simulink model "MDCC"  (R2021b)
settings: Solver=FixedStepDiscrete  StartTime=0.0  StopTime=10.0  FixedStep=0.0001  RelTol=1e-3
model workspace (MATLAB code in the model file):
  | cmdLim = Simulink.Parameter;
  | cmdLim.Value = 15;
  | cmdLim.Description = 'Limit for controlling the maximum surface command angle.';
  | cmdLim.Min = 0;
  | cmdLim.Max = 90;
  | cmdLim.DocUnits = 'deg';
  | 
  | dispGain = Simulink.Parameter;
  | dispGain.Value = 0.75;
  | dispGain.Description = 'Gain applied to the displacement error.';
  | dispGain.Min = 0;
  | dispGain.Max = [];
  | dispGain.DocUnits = 'deg/sec/deg';
  | 
  | dispLim = Simulink.Parameter;
  | dispLim.Value = 30;
  | dispLim.Description = 'Limit for controlling the maximum commanded angle.';
  | dispLim.Min = 0;
  | dispLim.Max = 180;
  | dispLim.DocUnits = 'deg';
  | 
  | intGain = Simulink.Parameter;
  | intGain.Value = 0.5;
  | intGain.Description = 'Gain applied to the integral error.';
  | intGain.Min = 0;
  | intGain.Max = [];
  | intGain.DocUnits = 'deg/sec/deg/sec';
  | 
  | intLim = Simulink.Parameter;
  | intLim.Value = 5;
  | intLim.Description = 'Limit for controlling the maximum commanded angle.';
  | intLim.Min = 0;
  | intLim.Max = 90;
  | intLim.DocUnits = 'deg';
  | 
  | rateGain = Simulink.Parameter;
  | rateGain.Value = 2;
  | rateGain.Description = 'Gain applied to the rate error.';
  | rateGain.Min = 0;
  | rateGain.Max = [];
  | rateGain.DocUnits = 'deg/deg/sec';
  | 
  | rateLim = Simulink.Parameter;
  | rateLim.Value = 6;
  | rateLim.Description = 'Limit for controlling the maximum commanded angle.';
  | rateLim.Min = 0;
  | rateLim.Max = 180;
  | rateLim.DocUnits = 'deg/sec';
  | 
  | hdgGain = Simulink.Parameter;
  | hdgGain.Value = 0.015;
values from neighbouring files (symbols this model uses):
  KfDeadCompen_SetDeltaTime_us = myPackage.Parameter    [DeadCompen.m]
  Ts = 5E-6    (= 5e-06)    [iPMSM_data.m]
  VbDeadComp_SwtUseIsttrDes_flg = myPackage.Parameter    [DeadCompen.m]
  VfDeadCompen_ISttrDdeThdSwt_A = myPackage.Parameter    [DeadCompen.m]
  VfDeadCompen_ISttrIgbtThdSwt_A = myPackage.Parameter    [DeadCompen.m]
  VfDeadCompen_rDdeISttrHi_R = myPackage.Parameter    [DeadCompen.m]
  VfDeadCompen_rDdeISttrLo_R = myPackage.Parameter    [DeadCompen.m]
  VfDeadCompen_rIgbtISttrHi_R = myPackage.Parameter    [DeadCompen.m]
  VfDeadCompen_rIgbtISttrLo_R = myPackage.Parameter    [DeadCompen.m]
  VfDeadCompen_uDdeISttrHi_V = myPackage.Parameter    [DeadCompen.m]
  VfDeadCompen_uDdeISttrLo_V = myPackage.Parameter    [DeadCompen.m]
  VfDeadCompen_uIgbtISttrHi_V = myPackage.Parameter    [DeadCompen.m]
  VfDeadCompen_uIgbtISttrLo_V = myPackage.Parameter    [DeadCompen.m]
undefined symbols (not defined in the file or in its folder): CosTable12bit_Y, GLBCal_GLBCal_Kf_DCLinkOverVolErrThd_V, GLBCal_GLBCal_Kf_DCLinkUnderVolErrThd_V, GLBCal_GLBCal_Kf_EquiLd_NULL, GLBCal_GLBCal_Kf_EquiLq_NULL, GLBCal_GLBCal_Kf_MotorRatedSpeed_rpm, GLBCal_GLBCal_Kf_MotorSpeedHysteresis_Coef, GLBCal_Ke_MotorPolePairsNum_NULL, IoHwAbOpArg_PwmDutyCyclePhU_NULL, IoHwAbOpArg_PwmDutyCyclePhV_NULL, IoHwAbOpArg_PwmDutyCyclePhW_NULL, IoHwAbOpArg_PwmOutputEn, KbMDCC_DeadTimeCompEn_flg, KbMDCC_MCF_flgHarmInIsdqTab11ZR_flg, KbMDCC_MCF_flgHarmInIsdqTab13ZR_flg, KbMDCC_MCF_flgHarmInIsdqTab5ZR_flg, KbMDCC_MCF_flgHarmInIsdqTab7ZR_flg, KbMDCC_MCF_flgHarmInject_flg, KbMDCC_SetEAngleEn_flg, KbMDCC_UdUqFwOmit_flg, KfDeadCompen_CpPeriodTimesT_NULL, KfMDCC_ActiveDischargeIdCurVal_A, KfMDCC_ActiveDischargeIqCurVal_A, KfMDCC_DCLinkVolRate_coef, KfMDCC_DebugEAngleInit_rad, KfMDCC_DebugUalphaVolCmd_V, KfMDCC_DebugUbetaVolCmd_V, KfMDCC_DebugUdCmd_V, KfMDCC_DebugUqCmd_V, KfMDCC_DebugUsCmd_V, KfMDCC_DebugUsRate_V, KfMDCC_IMCResp_NULL, KfMDCC_IMCStab_NULL, KfMDCC_InvParkCpPeriodTimesT_NULL, KfMDCC_MCF_CircAge_NULL, KfMDCC_MCF_flgUse11Harm_flg, KfMDCC_MCF_flgUse13Harm_flg, KfMDCC_MCF_flgUse5Harm_flg, KfMDCC_MCF_flgUse7Harm_flg, KfMDCC_MCF_Harm1113FLParamSpeedThrd_rads, KfMDCC_MCF_Harm57FLParamSpeedThrd_rads, KfMDCC_MCF_HarmcofFltN_NULL, KfMDCC_MCF_HarmCpnAg_NULL, KfMDCC_MCF_HarmfLParaHigh_coef, KfMDCC_MCF_HarmfLParaLow_coef, KfMDCC_MCF_HarmIn1113ZRY_Trq_Nm, KfMDCC_MCF_HarmIn11_SpdLimHigh_rads, KfMDCC_MCF_HarmIn11_SpdLimLow_rads, KfMDCC_MCF_HarmIn11ZRY_Isd_A, KfMDCC_MCF_HarmIn11ZRY_Isq_A, KfMDCC_MCF_HarmIn13_SpdLimHigh_rads, KfMDCC_MCF_HarmIn13_SpdLimLow_rads, KfMDCC_MCF_HarmIn13ZRY_Isd_A, KfMDCC_MCF_HarmIn13ZRY_Isq_A, KfMDCC_MCF_HarmIn57ZRY_Trq_Nm, KfMDCC_MCF_HarmIn5_SpdLimHigh_rads, KfMDCC_MCF_HarmIn5_SpdLimLow_rads, KfMDCC_MCF_HarmIn5ZRY_Isd_A, KfMDCC_MCF_HarmIn5ZRY_Isq_A, KfMDCC_MCF_HarmIn7_SpdLimHigh_rads ... (+47)
libraries: simulink x40, PMSM_Library x3, mcbcontrolslib x1
(part 4 of 8)

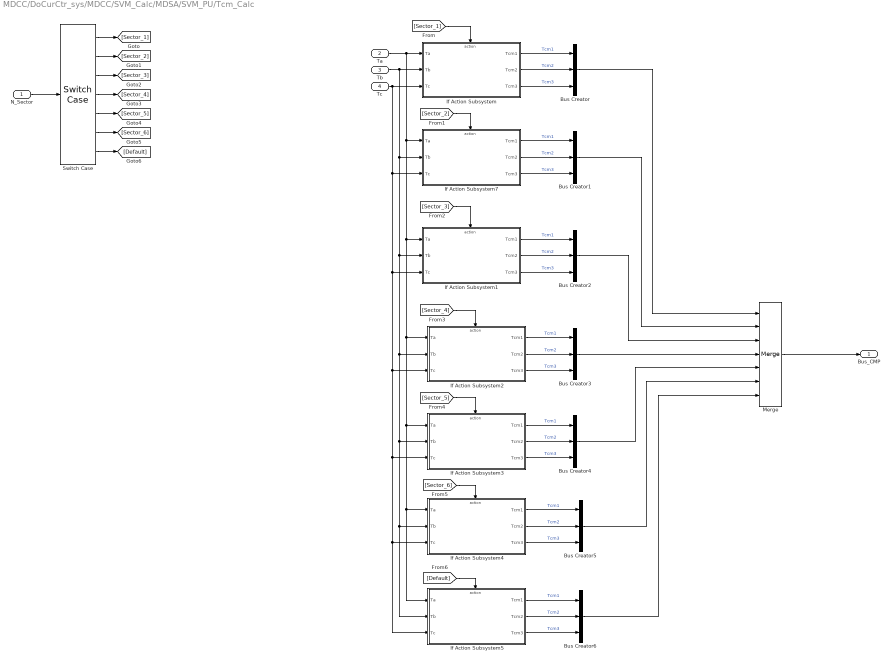
== system MDCC/DoCurCtr_sys/MDCC/SVM_Calc/MDSA/SVM_PU/Tcm_Calc ==
  N_Sector : Inport
  Ta : Inport  Port=2
  Tb : Inport  Port=3
  Tc : Inport  Port=4
  Bus Creator{,1..6} (7 alike) : BusCreator  Inputs=3
  If Action Subsystem : Subsystem  TreatAsAtomicUnit=on
  If Action Subsystem1 : Subsystem  TreatAsAtomicUnit=on
  If Action Subsystem2 : Subsystem  TreatAsAtomicUnit=on
  If Action Subsystem3 : Subsystem  TreatAsAtomicUnit=on
  If Action Subsystem4 : Subsystem  TreatAsAtomicUnit=on
  If Action Subsystem5 : Subsystem  TreatAsAtomicUnit=on
  If Action Subsystem7 : Subsystem  TreatAsAtomicUnit=on
  Merge : Merge  Inputs=7
  Switch Case : SwitchCase  CaseConditions={1,2,3,4,5,6}
  Bus_CMP : Outport
  wires:
  Switch Case/1 -> [Sector_1]
  Switch Case/2 -> [Sector_2]
  Switch Case/4 -> [Sector_4]
  Switch Case/6 -> [Sector_6]
  Switch Case/3 -> [Sector_3]
  N_Sector/1 -> Switch Case/1
  Switch Case/7 -> [Default]
  Switch Case/5 -> [Sector_5]
  [Sector_1] -> If Action Subsystem/Action
  [Sector_2] -> If Action Subsystem7/Action
  [Sector_4] -> If Action Subsystem2/Action
  [Sector_3] -> If Action Subsystem1/Action
  [Sector_6] -> If Action Subsystem4/Action
  [Sector_5] -> If Action Subsystem3/Action
  [Default] -> If Action Subsystem5/Action
  Tb/1 -> If Action Subsystem5/2(Tb), If Action Subsystem4/2(Tb), If Action Subsystem3/2(Tb), If Action Subsystem2/2(Tb), If Action Subsystem1/2(Tb), If Action Subsystem7/2(Tb), If Action Subsystem/2(Tb)
  Tc/1 -> If Action Subsystem/3(Tc), If Action Subsystem5/3(Tc), If Action Subsystem4/3(Tc), If Action Subsystem3/3(Tc), If Action Subsystem2/3(Tc), If Action Subsystem1/3(Tc), If Action Subsystem7/3(Tc)
  Ta/1 -> If Action Subsystem5/1(Ta), If Action Subsystem4/1(Ta), If Action Subsystem3/1(Ta), If Action Subsystem2/1(Ta), If Action Subsystem1/1(Ta), If Action Subsystem7/1(Ta), If Action Subsystem/1(Ta)
  Merge/1 -> Bus_CMP/1
  If Action Subsystem/1(Tcm1) -> Bus Creator/1  "Tcm1"
  If Action Subsystem/2(Tcm2) -> Bus Creator/2  "Tcm2"
  If Action Subsystem/3(Tcm3) -> Bus Creator/3  "Tcm3"
  If Action Subsystem7/1(Tcm1) -> Bus Creator1/1  "Tcm1"
  If Action Subsystem7/3(Tcm3) -> Bus Creator1/3  "Tcm3"
  If Action Subsystem7/2(Tcm2) -> Bus Creator1/2  "Tcm2"
  If Action Subsystem1/1(Tcm1) -> Bus Creator2/1  "Tcm1"
  If Action Subsystem1/3(Tcm3) -> Bus Creator2/3  "Tcm3"
  If Action Subsystem1/2(Tcm2) -> Bus Creator2/2  "Tcm2"
  If Action Subsystem2/1(Tcm1) -> Bus Creator3/1  "Tcm1"
  If Action Subsystem2/3(Tcm3) -> Bus Creator3/3  "Tcm3"
  If Action Subsystem2/2(Tcm2) -> Bus Creator3/2  "Tcm2"
  If Action Subsystem3/1(Tcm1) -> Bus Creator4/1  "Tcm1"
  If Action Subsystem3/3(Tcm3) -> Bus Creator4/3  "Tcm3"
  If Action Subsystem3/2(Tcm2) -> Bus Creator4/2  "Tcm2"
  If Action Subsystem4/1(Tcm1) -> Bus Creator5/1  "Tcm1"
  If Action Subsystem4/3(Tcm3) -> Bus Creator5/3  "Tcm3"
  If Action Subsystem4/2(Tcm2) -> Bus Creator5/2  "Tcm2"
  If Action Subsystem5/1(Tcm1) -> Bus Creator6/1  "Tcm1"
  If Action Subsystem5/3(Tcm3) -> Bus Creator6/3  "Tcm3"
  If Action Subsystem5/2(Tcm2) -> Bus Creator6/2  "Tcm2"
  Bus Creator/1 -> Merge/1
  Bus Creator1/1 -> Merge/2
  Bus Creator2/1 -> Merge/3
  Bus Creator3/1 -> Merge/4
  Bus Creator4/1 -> Merge/5
  Bus Creator5/1 -> Merge/6
  Bus Creator6/1 -> Merge/7

== system MDCC/DoCurCtr_sys/MDCC/SVM_Calc/MDSA/SVPWM/vIntp_PWMFOC_CalSec ==
  Bus_UalphaUbeta : Inport
  CalABC : Subsystem
  CalSecValue : Subsystem
  CalVaVbVc : Subsystem  TreatAsAtomicUnit=on
  SecValue : Outport
  N_VALUE : Outport  Port=2
  wires:
  CalSecValue/2(N_VALUE) -> N_VALUE/1
  Bus_UalphaUbeta/1 -> CalVaVbVc/1(Bus_UalphaUbeta)
  CalSecValue/1(SecValue) -> SecValue/1
  CalABC/1(Bus_ABC) -> CalSecValue/1(Bus_ABC_IN)
  CalVaVbVc/1(Bus_Vabc) -> CalABC/1(Bus_Vabc_IN)

== system MDCC/DoCurCtr_sys/MDCC/SVM_Calc/MDSA/SVPWM/vIntp_PWMFOC_CalTriCompValue ==
  note: // 需要确定PWM的passive level
  N_VALUE_IN : Inport
  Bus_UalphaUbeta : Inport  Port=2
  Bus_Ts_Vdc : Inport  Port=3
  CalCMPValue : Subsystem
  CalTabc : Subsystem
  CalXYZ : Subsystem
  Bus_CMP : Outport
  wires:
  Bus_Ts_Vdc/1 -> CalXYZ/2(Bus_Ts_Vdc), CalTabc/2(Bus_Ts_Vdc)
  CalCMPValue/1(Bus_CMP) -> Bus_CMP/1
  CalTabc/1(Bus_Tabc) -> CalCMPValue/1(Bus_Tabc_IN)
  CalXYZ/1(BUS_XYZ) -> CalTabc/1(Bus_XYZ_IN)
  Bus_UalphaUbeta/1 -> CalXYZ/1(Bus_UalphaUbeta)
  N_VALUE_IN/1 -> CalCMPValue/2(N_VALUE_IN), CalTabc/3(N_VALUE_IN)

== system MDCC/DoCurCtr_sys/MDCC/UdUqCalc_Sys/MDCC_MCF_Sys/Enabled Subsystem/Harmonic_Injection_11 ==
  note: 扭矩滞环
  TDC_TrqDes : Inport
  MCF_Harm_isdAct11 : Inport  Port=2
  MCF_Harm_isqAct11 : Inport  Port=3
  MCF_Sin11Ag : Inport  Port=4
  MCF_Cos11Ag : Inport  Port=5
  Rdc_absnWoFlt_rads : Inport  Port=6
  MCF_uDcLnk : Inport  Port=7
  Bus Creator : BusCreator  Inputs=2
  Bus Creator1 : BusCreator  Inputs=2
  Bus Selector : BusSelector  OutputSignals=MCF_uAlpha_Harm11,MCF_uBeta_Harm11
  Set_11_steps_current_isdqdes : Subsystem
  Signal Copy : SignalConversion  OverrideOpt=off
  Signal Copy1 : SignalConversion  OverrideOpt=off
  Subsystem : Subsystem
  Subsystem1 : Subsystem
  Subsystem2 : Subsystem
  Switch2 : Switch  Criteria=u2 ~= 0
  Unit Delay : UnitDelay  SampleTime=-1  HasFrameUpgradeWarning=on
  Zero : Constant  Value=0  OutDataTypeStr=single
  Zero1 : Constant  Value=0  OutDataTypeStr=single
  MCF_uAlpha_Harm11 : Outport
  MCF_uBeta_Harm11 : Outport  Port=2
  wires:
  Bus Selector/2 -> Signal Copy1/1  "<MCF_uBeta_Harm11>"
  Subsystem/1(MCF_uAlpha_Harm11) -> Bus Creator/1  "MCF_uAlpha_Harm11"
  Zero1/1 -> Bus Creator1/2  "MCF_uBeta_Harm11"
  Switch2/1 -> Bus Selector/1
  Bus Creator/1 -> Switch2/1
  Bus Creator1/1 -> Switch2/3
  Zero/1 -> Bus Creator1/1  "MCF_uAlpha_Harm11"
  Subsystem/2(MCF_uBeta_Harm11) -> Bus Creator/2  "MCF_uBeta_Harm11"
  Bus Selector/1 -> Signal Copy/1  "<MCF_uAlpha_Harm11>"
  Subsystem1/1(Out2) -> Subsystem/Enable, Switch2/2, [flgHarmUse], Unit Delay/1
  Signal Copy/1 -> MCF_uAlpha_Harm11/1  "VAR_MCF_uAlpha_Harm11_f32"
  Signal Copy1/1 -> MCF_uBeta_Harm11/1  "VAR_MCF_uBeta_Harm11_f32"
  MCF_Harm_isdAct11/1 -> Subsystem/3(MCF_Harm_isdAct11)
  MCF_Harm_isqAct11/1 -> Subsystem/4(MCF_Harm_isqAct11)
  Unit Delay/1 -> Subsystem/8(MCF_flgHarm11PIRest)
  MCF_Sin11Ag/1 -> Subsystem/5(MCF_Sin11Ag)
  MCF_Cos11Ag/1 -> Subsystem/6(MCF_Cos11Ag)
  Rdc_absnWoFlt_rads/1 -> Subsystem1/1(Rdc_absnWoFlt_rads), Subsystem/7(Rdc_absnWoFlt_rads)
  Set_11_steps_current_isdqdes/1(VfMDCC_MCF_IsdDes11Harm_A) -> Subsystem/1(MCF_Harm_isdDes11)
  Set_11_steps_current_isdqdes/2(VfMDCC_MCF_IsqDes11Harm_A) -> Subsystem/2(MCF_Harm_isqDes11)
  TDC_TrqDes/1 -> Subsystem2/1(TDC_TrqDes)
  Subsystem2/1(TDC_TrqDesFlt) -> Set_11_steps_current_isdqdes/1(TDC_TrqDesFlt)
  [flgHarmUse] -> Subsystem2/2(flgHarmUse)
  MCF_uDcLnk/1 -> Subsystem1/2(MCF_uDcLnk)

== system MDCC/DoCurCtr_sys/MDCC/UdUqCalc_Sys/MDCC_MCF_Sys/Enabled Subsystem/Harmonic_Injection_13 ==
  note: 扭矩滞环
  TDC_TrqDes : Inport
  MCF_Harm_isdAct13 : Inport  Port=2
  MCF_Harm_isqAct13 : Inport  Port=3
  MCF_Sin13Ag : Inport  Port=4
  MCF_Cos13Ag : Inport  Port=5
  Rdc_absnWoFlt_rads : Inport  Port=6
  MCF_uDcLnk : Inport  Port=7
  Bus Creator : BusCreator  Inputs=2
  Bus Creator1 : BusCreator  Inputs=2
  Bus Selector : BusSelector  OutputSignals=MCF_uAlpha_Harm13,MCF_uBeta_Harm13
  Set_13_steps_current_isdqdes : Subsystem
  Signal Copy : SignalConversion  OverrideOpt=off
  Signal Copy1 : SignalConversion  OverrideOpt=off
  Subsystem : Subsystem
  Subsystem1 : Subsystem
  Subsystem2 : Subsystem
  Switch2 : Switch  Criteria=u2 ~= 0
  Unit Delay : UnitDelay  SampleTime=-1  HasFrameUpgradeWarning=on
  Zero : Constant  Value=0  OutDataTypeStr=single
  Zero1 : Constant  Value=0  OutDataTypeStr=single
  MCF_uAlpha_Harm13 : Outport
  MCF_uBeta_Harm13 : Outport  Port=2
  wires:
  Bus Selector/2 -> Signal Copy1/1  "<MCF_uBeta_Harm13>"
  Subsystem/1(MCF_uAlpha_Harm13) -> Bus Creator/1  "MCF_uAlpha_Harm13"
  Zero1/1 -> Bus Creator1/2  "MCF_uBeta_Harm13"
  Switch2/1 -> Bus Selector/1
  Bus Creator/1 -> Switch2/1
  Bus Creator1/1 -> Switch2/3
  Zero/1 -> Bus Creator1/1  "MCF_uAlpha_Harm13"
  Subsystem/2(MCF_uBeta_Harm13) -> Bus Creator/2  "MCF_uBeta_Harm13"
  Bus Selector/1 -> Signal Copy/1  "<MCF_uAlpha_Harm13>"
  Subsystem1/1(Out2) -> Subsystem/Enable, Switch2/2, [flgHarmUse], Unit Delay/1
  Signal Copy/1 -> MCF_uAlpha_Harm13/1  "VAR_MCF_uAlpha_Harm13_f32"
  Signal Copy1/1 -> MCF_uBeta_Harm13/1  "VAR_MCF_uBeta_Harm13_f32"
  MCF_Harm_isdAct13/1 -> Subsystem/3(MCF_Harm_isdAct13)
  MCF_Harm_isqAct13/1 -> Subsystem/4(MCF_Harm_isqAct13)
  Unit Delay/1 -> Subsystem/8(MCF_flgHarm13PIRest)
  MCF_Sin13Ag/1 -> Subsystem/5(MCF_Sin13Ag)
  MCF_Cos13Ag/1 -> Subsystem/6(MCF_Cos13Ag)
  Rdc_absnWoFlt_rads/1 -> Subsystem1/1(Rdc_absnWoFlt_rads), Subsystem/7(Rdc_absnWoFlt_rads)
  Set_13_steps_current_isdqdes/1(VfMDCC_MCF_IsdDes13Harm_A) -> Subsystem/1(MCF_Harm_isdDes13)
  Set_13_steps_current_isdqdes/2(VfMDCC_MCF_IsqDes13Harm_A) -> Subsystem/2(MCF_Harm_isqDes13)
  TDC_TrqDes/1 -> Subsystem2/1(TDC_TrqDes)
  Subsystem2/1(TDC_TrqDesFlt) -> Set_13_steps_current_isdqdes/1(TDC_TrqDesFlt)
  [flgHarmUse] -> Subsystem2/2(flgHarmUse)
  MCF_uDcLnk/1 -> Subsystem1/2(MCF_uDcLnk)

== system MDCC/DoCurCtr_sys/MDCC/UdUqCalc_Sys/MDCC_MCF_Sys/Enabled Subsystem/Harmonic_Injection_5 ==
  note: 扭矩滞环
  TDC_TrqDes : Inport
  MCF_Harm_isdAct5 : Inport  Port=2
  MCF_Harm_isqAct5 : Inport  Port=3
  MCF_Sin5Ag : Inport  Port=4
  MCF_Cos5Ag : Inport  Port=5
  Rdc_absnWoFlt_rads : Inport  Port=6
  MCF_uDcLnk : Inport  Port=7
  Bus Creator : BusCreator  Inputs=2
  Bus Creator1 : BusCreator  Inputs=2
  Bus Selector : BusSelector  OutputSignals=MCF_uAlpha_Harm5,MCF_uBeta_Harm5
  Set_5_steps_current_isdqdes : Subsystem
  Signal Copy : SignalConversion  OverrideOpt=off
  Signal Copy1 : SignalConversion  OverrideOpt=off
  Subsystem : Subsystem
  Subsystem1 : Subsystem
  Subsystem2 : Subsystem
  Switch2 : Switch  Criteria=u2 ~= 0
  Unit Delay : UnitDelay  SampleTime=-1  HasFrameUpgradeWarning=on
  Zero : Constant  Value=0  OutDataTypeStr=single
  Zero1 : Constant  Value=0  OutDataTypeStr=single
  MCF_uAlpha_Harm5 : Outport
  MCF_uBeta_Harm5 : Outport  Port=2
  wires:
  Bus Selector/2 -> Signal Copy1/1  "<MCF_uBeta_Harm5>"
  Subsystem/1(MCF_uAlpha_Harm5) -> Bus Creator/1  "MCF_uAlpha_Harm5"
  Zero1/1 -> Bus Creator1/2  "MCF_uBeta_Harm5"
  Switch2/1 -> Bus Selector/1
  Bus Creator/1 -> Switch2/1
  Bus Creator1/1 -> Switch2/3
  Zero/1 -> Bus Creator1/1  "MCF_uAlpha_Harm5"
  Subsystem/2(MCF_uBeta_Harm5) -> Bus Creator/2  "MCF_uBeta_Harm5"
  Bus Selector/1 -> Signal Copy/1  "<MCF_uAlpha_Harm5>"
  Subsystem1/1(Out2) -> Subsystem/Enable, Switch2/2, [flgHarmUse], Unit Delay/1
  Signal Copy/1 -> MCF_uAlpha_Harm5/1  "VAR_MCF_uAlpha_Harm5_f32"
  Signal Copy1/1 -> MCF_uBeta_Harm5/1  "VAR_MCF_uBeta_Harm5_f32"
  MCF_Harm_isdAct5/1 -> Subsystem/3(MCF_Harm_isdAct5)
  MCF_Harm_isqAct5/1 -> Subsystem/4(MCF_Harm_isqAct5)
  Unit Delay/1 -> Subsystem/8(MCF_flgHarm5PIRest)
  MCF_Sin5Ag/1 -> Subsystem/5(MCF_Sin5Ag)
  MCF_Cos5Ag/1 -> Subsystem/6(MCF_Cos5Ag)
  Rdc_absnWoFlt_rads/1 -> Subsystem1/1(Rdc_absnWoFlt_rads), Subsystem/7(Rdc_absnWoFlt_rads)
  Set_5_steps_current_isdqdes/1(VfMDCC_MCF_IsdDes5Harm_A) -> Subsystem/1(MCF_Harm_isdDes5)
  Set_5_steps_current_isdqdes/2(VfMDCC_MCF_IsqDes5Harm_A) -> Subsystem/2(MCF_Harm_isqDes5)
  TDC_TrqDes/1 -> Subsystem2/1(TDC_TrqDes)
  Subsystem2/1(TDC_TrqDesFlt) -> Set_5_steps_current_isdqdes/1(TDC_TrqDesFlt)
  [flgHarmUse] -> Subsystem2/2(flgHarmUse)
  MCF_uDcLnk/1 -> Subsystem1/2(MCF_uDcLnk)

== system MDCC/DoCurCtr_sys/MDCC/UdUqCalc_Sys/MDCC_MCF_Sys/Enabled Subsystem/Harmonic_Injection_7 ==
  note: 扭矩滞环
  TDC_TrqDes : Inport
  MCF_Harm_isdAct7 : Inport  Port=2
  MCF_Harm_isqAct7 : Inport  Port=3
  MCF_Sin7Ag : Inport  Port=4
  MCF_Cos7Ag : Inport  Port=5
  Rdc_absnWoFlt_rads : Inport  Port=6
  MCF_uDcLnk : Inport  Port=7
  Bus Creator : BusCreator  Inputs=2
  Bus Creator1 : BusCreator  Inputs=2
  Bus Selector : BusSelector  OutputSignals=MCF_uAlpha_Harm7,MCF_uBeta_Harm7
  Set_7_steps_current_isdqdes : Subsystem
  Signal Copy : SignalConversion  OverrideOpt=off
  Signal Copy1 : SignalConversion  OverrideOpt=off
  Subsystem : Subsystem
  Subsystem1 : Subsystem
  Subsystem2 : Subsystem
  Switch2 : Switch  Criteria=u2 ~= 0
  Unit Delay : UnitDelay  SampleTime=-1  HasFrameUpgradeWarning=on
  Zero : Constant  Value=0  OutDataTypeStr=single
  Zero1 : Constant  Value=0  OutDataTypeStr=single
  MCF_uAlpha_Harm7 : Outport
  MCF_uBeta_Harm7 : Outport  Port=2
  wires:
  Bus Selector/2 -> Signal Copy1/1  "<MCF_uBeta_Harm7>"
  Subsystem/1(MCF_uAlpha_Harm7) -> Bus Creator/1  "MCF_uAlpha_Harm7"
  Zero1/1 -> Bus Creator1/2  "MCF_uBeta_Harm7"
  Switch2/1 -> Bus Selector/1
  Bus Creator/1 -> Switch2/1
  Bus Creator1/1 -> Switch2/3
  Zero/1 -> Bus Creator1/1  "MCF_uAlpha_Harm7"
  Subsystem/2(MCF_uBeta_Harm7) -> Bus Creator/2  "MCF_uBeta_Harm7"
  Bus Selector/1 -> Signal Copy/1  "<MCF_uAlpha_Harm7>"
  Subsystem1/1(Out2) -> Subsystem/Enable, Switch2/2, [flgHarmUse], Unit Delay/1
  Signal Copy/1 -> MCF_uAlpha_Harm7/1  "VAR_MCF_uAlpha_Harm7_f32"
  Signal Copy1/1 -> MCF_uBeta_Harm7/1  "VAR_MCF_uBeta_Harm7_f32"
  MCF_Harm_isdAct7/1 -> Subsystem/3(MCF_Harm_isdAct7)
  MCF_Harm_isqAct7/1 -> Subsystem/4(MCF_Harm_isqAct7)
  Unit Delay/1 -> Subsystem/8(MCF_flgHarm7PIRest)
  MCF_Sin7Ag/1 -> Subsystem/5(MCF_Sin7Ag)
  MCF_Cos7Ag/1 -> Subsystem/6(MCF_Cos7Ag)
  Rdc_absnWoFlt_rads/1 -> Subsystem1/1(Rdc_absnWoFlt_rads), Subsystem/7(Rdc_absnWoFlt_rads)
  Set_7_steps_current_isdqdes/1(VfMDCC_MCF_IsdDes7Harm_A) -> Subsystem/1(MCF_Harm_isdDes7)
  Set_7_steps_current_isdqdes/2(VfMDCC_MCF_IsqDes7Harm_A) -> Subsystem/2(MCF_Harm_isqDes7)
  TDC_TrqDes/1 -> Subsystem2/1(TDC_TrqDes)
  Subsystem2/1(TDC_TrqDesFlt) -> Set_7_steps_current_isdqdes/1(TDC_TrqDesFlt)
  [flgHarmUse] -> Subsystem2/2(flgHarmUse)
  MCF_uDcLnk/1 -> Subsystem1/2(MCF_uDcLnk)

== system MDCC/DoCurCtr_sys/MDCC/UdUqCalc_Sys/MDCC_MCF_Sys/Enabled Subsystem/Subsystem1 ==
  VfMDCC_AlphaCurHarmonic_A : Inport
  VfMDCC_BetaCurHarmonic_A : Inport  Port=2
  VuMDCC_MotorPositionCnt_NULL : Inport  Port=3
  VfMDTM_PwmCycleTime_s : Inport  Port=4
  VfMDSP_MotorESpeed_rads : Inport  Port=5
  Compare To Constant : simulink/Logic and Bit Operations/Compare To Constant  relop=<=  const=KfMDCC_MCF_Harm57FLParamSpeedThrd_rads  OutDataTypeStr=boolean
  Compare To Constant1 : simulink/Logic and Bit Operations/Compare To Constant  relop=<=  const=KfMDCC_MCF_Harm1113FLParamSpeedThrd_rads  OutDataTypeStr=boolean
  Constant1 : Constant  Value=KfMDCC_MCF_HarmfLParaLow_coef  OutDataTypeStr=single
  Constant3 : Constant  Value=KfMDCC_MCF_HarmfLParaHigh_coef  OutDataTypeStr=single
  Park11 : Subsystem  TreatAsAtomicUnit=on  RTWFcnName=Harm_Park_Calc
      settings: RTWFcnNameOpts=User specified
  Park13 : Subsystem  TreatAsAtomicUnit=on  RTWFcnName=Harm_Park_Calc
      settings: RTWFcnNameOpts=User specified
  Park5 : Subsystem  TreatAsAtomicUnit=on  RTWFcnName=Harm_Park_Calc
      settings: RTWFcnNameOpts=User specified
  Park7 : Subsystem  TreatAsAtomicUnit=on  RTWFcnName=Harm_Park_Calc
      settings: RTWFcnNameOpts=User specified
  Subsystem : Subsystem
  Switch : Switch  Criteria=u2 ~= 0
  Switch1 : Switch  Criteria=u2 ~= 0
  MCF_Id5_Harm : Outport
  MCF_Iq5_Harm : Outport  Port=2
  MCF_Id7_Harm : Outport  Port=3
  MCF_Iq7_Harm : Outport  Port=4
  MCF_Id11_Harm : Outport  Port=5
  MCF_Iq11_Harm : Outport  Port=6
  MCF_Id13_Harm : Outport  Port=7
  MCF_Iq13_Harm : Outport  Port=8
  wires:
  Subsystem/5(MCF_AgSin11) -> Park11/1(MCF_AgSin)
  VfMDCC_AlphaCurHarmonic_A/1 -> Park13/2(MCF_ialpha_Harm), Park11/2(MCF_ialpha_Harm), Park7/2(MCF_ialpha_Harm), Park5/2(MCF_ialpha_Harm)
  Constant1/1 -> Switch/1, Switch1/1
  Park7/1(MCF_Id_Harm) -> MCF_Id7_Harm/1
  [dB_Harm1113] -> Park11/6(dB_Harm), Park13/6(dB_Harm)
  Switch1/1 -> [dB_Harm1113]
  Subsystem/8(MCF_AgCos13) -> Park13/4(MCF_AgCos)
  VuMDCC_MotorPositionCnt_NULL/1 -> Subsystem/1(VuMDCC_MotorPositionCnt_NULL)
  VfMDTM_PwmCycleTime_s/1 -> Park13/5(MCF_dtPWM), Park11/5(MCF_dtPWM), Park7/5(MCF_dtPWM), Park5/5(MCF_dtPWM)
  Subsystem/4(MCF_AgCos7) -> Park7/4(MCF_AgCos)
  Compare To Constant1/1 -> Switch1/2
  Subsystem/3(MCF_AgSin7) -> Park7/1(MCF_AgSin)
  VfMDSP_MotorESpeed_rads/1 -> Compare To Constant/1, Compare To Constant1/1
  VfMDCC_BetaCurHarmonic_A/1 -> Park13/3(MCF_ibeta_Harm), Park11/3(MCF_ibeta_Harm), Park7/3(MCF_ibeta_Harm), Park5/3(MCF_ibeta_Harm)
  Switch/1 -> [dB_Harm57]
  Subsystem/2(MCF_AgCos5) -> Park5/4(MCF_AgCos)
  Compare To Constant/1 -> Switch/2
  Park5/1(MCF_Id_Harm) -> MCF_Id5_Harm/1
  Subsystem/7(MCF_AgSin13) -> Park13/1(MCF_AgSin)
  [dB_Harm57] -> Park5/6(dB_Harm), Park7/6(dB_Harm)
  Subsystem/1(MCF_AgSin5) -> Park5/1(MCF_AgSin)
  Park13/2(MCF_Iq_Harm) -> MCF_Iq13_Harm/1
  Park13/1(MCF_Id_Harm) -> MCF_Id13_Harm/1
  Park11/2(MCF_Iq_Harm) -> MCF_Iq11_Harm/1
  Subsystem/6(MCF_AgCos11) -> Park11/4(MCF_AgCos)
  Park5/2(MCF_Iq_Harm) -> MCF_Iq5_Harm/1
  Constant3/1 -> Switch1/3, Switch/3
  Park7/2(MCF_Iq_Harm) -> MCF_Iq7_Harm/1
  Park11/1(MCF_Id_Harm) -> MCF_Id11_Harm/1

== system MDCC/DoCurCtr_sys/MDCC/UdUqCalc_Sys/MDCC_MCF_Sys/Enabled Subsystem/Subsystem2 ==
  VuMDCC_MotorPositionCnt_NULL : Inport
  VfMDTM_PwmCycleTime_s : Inport  Port=2
  VfMDSP_MotorESpeed_rads : Inport  Port=3
  Constant1 : Constant  Value=7  OutDataTypeStr=single
  Constant2 : Constant  Value=-5  OutDataTypeStr=single
  Constant3 : Constant  Value=-11  OutDataTypeStr=single
  Constant4 : Constant  Value=13  OutDataTypeStr=single
  Mcf_AgTranCalc11 : Subsystem
  Mcf_AgTranCalc13 : Subsystem
  Mcf_AgTranCalc5 : Subsystem
  Mcf_AgTranCalc7 : Subsystem
  Subsystem : Subsystem
  MCF_Harm5_SinAg : Outport
  MCF_Harm5_CosAg : Outport  Port=2
  MCF_Harm7_SinAg : Outport  Port=3
  MCF_Harm7_CosAg : Outport  Port=4
  MCF_Harm11_SinAg : Outport  Port=5
  MCF_Harm11_CosAg : Outport  Port=6
  MCF_Harm13_SinAg : Outport  Port=7
  MCF_Harm13_CosAg : Outport  Port=8
  wires:
  Mcf_AgTranCalc5/1(MCF_SinAg) -> MCF_Harm5_SinAg/1
  Mcf_AgTranCalc5/2(MCF_CosAg) -> MCF_Harm5_CosAg/1
  Mcf_AgTranCalc7/2(MCF_CosAg) -> MCF_Harm7_CosAg/1
  Mcf_AgTranCalc7/1(MCF_SinAg) -> MCF_Harm7_SinAg/1
  Mcf_AgTranCalc11/1(MCF_SinAg) -> MCF_Harm11_SinAg/1
  Mcf_AgTranCalc11/2(MCF_CosAg) -> MCF_Harm11_CosAg/1
  Mcf_AgTranCalc13/1(MCF_SinAg) -> MCF_Harm13_SinAg/1
  Mcf_AgTranCalc13/2(MCF_CosAg) -> MCF_Harm13_CosAg/1
  VfMDTM_PwmCycleTime_s/1 -> Subsystem/2(dtPwmWoRpwm)
  VfMDSP_MotorESpeed_rads/1 -> Subsystem/1(HSPF_nSlowFlt)
  Subsystem/1(Harm_AgCpn) -> Mcf_AgTranCalc7/1(Harm_AgCpn), Mcf_AgTranCalc13/1(Harm_AgCpn), Mcf_AgTranCalc11/1(Harm_AgCpn), Mcf_AgTranCalc5/1(Harm_AgCpn)
  VuMDCC_MotorPositionCnt_NULL/1 -> Subsystem/3(MCF_agRtrEe)
  Constant2/1 -> Mcf_AgTranCalc5/2(Harm_coef)
  Constant1/1 -> Mcf_AgTranCalc7/2(Harm_coef)
  Constant3/1 -> Mcf_AgTranCalc11/2(Harm_coef)
  Constant4/1 -> Mcf_AgTranCalc13/2(Harm_coef)

== system MDCC/DoCurCtr_sys/MDCC/UdUqCalc_Sys/MDCC_MCF_Sys/Subsystem/iU_SOGI ==
  MCF_iPhase : Inport
  MotorESpeed_rads : Inport  Port=2
  PwmCycleTime_s : Inport  Port=3
  Add : Sum  Inputs=-+
  Add1 : Sum  Inputs=+-
  Add2 : Sum
  Add3 : Sum
  Constant : Constant  OutDataTypeStr=single
  Divide : Product  Inputs=**
  Divide1 : Product  Inputs=**
  Divide2 : Product  Inputs=**
  Divide3 : Product  Inputs=*/  OutDataTypeStr=single
  Gain : Gain  Gain=1.414
  Unit Delay : UnitDelay  SampleTime=-1  HasFrameUpgradeWarning=on
  Unit Delay1 : UnitDelay  SampleTime=-1  HasFrameUpgradeWarning=on
  Unit Delay2 : UnitDelay  SampleTime=-1  HasFrameUpgradeWarning=on
  iPhaseBase_A : Outport
  wires:
  Add2/1 -> iPhaseBase_A/1, Divide1/2, Unit Delay1/1
  Divide/1 -> Add2/2
  Gain/1 -> Add1/1
  Add3/1 -> Unit Delay2/1
  Unit Delay2/1 -> Add3/1, Add1/2
  Unit Delay/1 -> Add/2
  Unit Delay1/1 -> Add2/1, Add/1
  Add/1 -> Gain/1
  Divide2/1 -> Divide1/1, Divide/2
  MCF_iPhase/1 -> Unit Delay/1
  MotorESpeed_rads/1 -> Divide2/1
  Divide1/1 -> Add3/2
  Divide3/1 -> Divide2/2
  Constant/1 -> Divide3/1
  Add1/1 -> Divide/1
  PwmCycleTime_s/1 -> Divide3/2

== system MDCC/DoCurCtr_sys/MDCC/UdUqCalc_Sys/MDCC_MCF_Sys/Subsystem/iV_SOGI ==
  MCF_iPhase : Inport
  MotorESpeed_rads : Inport  Port=2
  PwmCycleTime_s : Inport  Port=3
  Add : Sum  Inputs=-+
  Add1 : Sum  Inputs=+-
  Add2 : Sum
  Add3 : Sum
  Constant : Constant  OutDataTypeStr=single
  Divide : Product  Inputs=**
  Divide1 : Product  Inputs=**
  Divide2 : Product  Inputs=**
  Divide3 : Product  Inputs=*/  OutDataTypeStr=single
  Gain : Gain  Gain=1.414
  Unit Delay : UnitDelay  SampleTime=-1  HasFrameUpgradeWarning=on
  Unit Delay1 : UnitDelay  SampleTime=-1  HasFrameUpgradeWarning=on
  Unit Delay2 : UnitDelay  SampleTime=-1  HasFrameUpgradeWarning=on
  iPhaseBase_A : Outport
  wires:
  Add2/1 -> iPhaseBase_A/1, Divide1/2, Unit Delay1/1
  Divide/1 -> Add2/2
  Gain/1 -> Add1/1
  Add3/1 -> Unit Delay2/1
  Unit Delay2/1 -> Add3/1, Add1/2
  Unit Delay/1 -> Add/2
  Unit Delay1/1 -> Add2/1, Add/1
  Add/1 -> Gain/1
  Divide2/1 -> Divide1/1, Divide/2
  MCF_iPhase/1 -> Unit Delay/1
  MotorESpeed_rads/1 -> Divide2/1
  Divide1/1 -> Add3/2
  Divide3/1 -> Divide2/2
  Constant/1 -> Divide3/1
  Add1/1 -> Divide/1
  PwmCycleTime_s/1 -> Divide3/2

== system MDCC/DoCurCtr_sys/MDCC/UdUqCalc_Sys/MDCC_MCF_Sys/Subsystem/iW_SOGI ==
  MCF_iPhase : Inport
  MotorESpeed_rads : Inport  Port=2
  PwmCycleTime_s : Inport  Port=3
  Add : Sum  Inputs=-+
  Add1 : Sum  Inputs=+-
  Add2 : Sum
  Add3 : Sum
  Constant : Constant  OutDataTypeStr=single
  Divide : Product  Inputs=**
  Divide1 : Product  Inputs=**
  Divide2 : Product  Inputs=**
  Divide3 : Product  Inputs=*/  OutDataTypeStr=single
  Gain : Gain  Gain=1.414
  Unit Delay : UnitDelay  SampleTime=-1  HasFrameUpgradeWarning=on
  Unit Delay1 : UnitDelay  SampleTime=-1  HasFrameUpgradeWarning=on
  Unit Delay2 : UnitDelay  SampleTime=-1  HasFrameUpgradeWarning=on
  iPhaseBase_A : Outport
  wires:
  Add2/1 -> iPhaseBase_A/1, Divide1/2, Unit Delay1/1
  Divide/1 -> Add2/2
  Gain/1 -> Add1/1
  Add3/1 -> Unit Delay2/1
  Unit Delay2/1 -> Add3/1, Add1/2
  Unit Delay/1 -> Add/2
  Unit Delay1/1 -> Add2/1, Add/1
  Add/1 -> Gain/1
  Divide2/1 -> Divide1/1, Divide/2
  MCF_iPhase/1 -> Unit Delay/1
  MotorESpeed_rads/1 -> Divide2/1
  Divide1/1 -> Add3/2
  Divide3/1 -> Divide2/2
  Constant/1 -> Divide3/1
  Add1/1 -> Divide/1
  PwmCycleTime_s/1 -> Divide3/2

== system MDCC/DoCurCtr_sys/MDCC/UdUqCalc_Sys/SelfHeating/Subsystem1/SinCounter_10ms ==
  CNT : Inport
  Add : Sum
  Constant1 : Constant  OutDataTypeStr=uint16
  Constant2 : Constant  Value=0  OutDataTypeStr=uint16
  Delay : Delay  DelayLength=1
  Relational Operator : RelationalOperator  Operator=<=  OutDataTypeStr=boolean  RndMeth=Simplest
  Switch : Switch  Criteria=u2 ~= 0
  En : Outport
  wires:
  Add/1 -> Relational Operator/2, Switch/3
  Relational Operator/1 -> Switch/2, En/1  "En"
  Delay/1 -> Add/2
  Constant1/1 -> Add/1
  Constant2/1 -> Switch/1
  Switch/1 -> Delay/1
  CNT/1 -> Relational Operator/1

== system MDCC/DoCurCtr_sys/MDCC/UdUqCalc_Sys/SelfHeating/Subsystem1/Subsystem ==
  VfMDTM_SelfHeatingEAngle_NULL : Inport
  VfMDTM_SelfHeatingUdVal_V_Set : Inport  Port=2
  Enable : EnablePort
  Constant3 : Constant  Value=SinTable12bit_Y
  Direct Lookup Table (n-D)1 : LookupNDDirect  NumberOfTableDimensions=1  TableIsInput=on  Table=[4 5 6]  TableMax=[4096]
  Product : Product
  VfMDTM_SelfHeatingUdVal_V : Outport
  wires:
  Constant3/1 -> Direct Lookup Table (n-D)1/2
  Direct Lookup Table (n-D)1/1 -> Product/1
  VfMDTM_SelfHeatingEAngle_NULL/1 -> Direct Lookup Table (n-D)1/1
  Product/1 -> VfMDTM_SelfHeatingUdVal_V/1
  VfMDTM_SelfHeatingUdVal_V_Set/1 -> Product/2

== system MDCC/DoCurCtr_sys/MDCC/UdUqCalc_Sys/SelfHeating/Subsystem1/Subsystem1 ==
  set : Inport
  rate : Inport  Port=2
  Enable : EnablePort
  Delay : Delay  DelayLength=1
  Relational Operator : RelationalOperator  Operator=<  OutDataTypeStr=boolean  RndMeth=Simplest
  Subsystem1 : Subsystem
  VfMDTM_SelfHeatingUdVal_V_Set : Outport
  VbMDCC_SelfHeatingStop_flg : Outport  Port=2
  wires:
  set/1 -> Subsystem1/1(set)
  Delay/1 -> Subsystem1/3(this_ref)
  Subsystem1/1(VfMDTM_SelfHeatingUdVal_V) -> VfMDTM_SelfHeatingUdVal_V_Set/1, Relational Operator/1, Delay/1
  rate/1 -> Relational Operator/2, Subsystem1/2(rate)
  Relational Operator/1 -> VbMDCC_SelfHeatingStop_flg/1

== system MDCC/DoCurCtr_sys/MDCC/UdUqCalc_Sys/SelfHeating/Subsystem1/Subsystem2 ==
  VfMDTM_SelfHeatingEAngle_NULL : Inport
  VfMDTM_SelfHeatingUdVal_V_Set : Inport  Port=2
  Enable : EnablePort
  Product : Product
  VfMDTM_SelfHeatingUdVal_V : Outport
  wires:
  VfMDTM_SelfHeatingEAngle_NULL/1 -> Product/1
  Product/1 -> VfMDTM_SelfHeatingUdVal_V/1
  VfMDTM_SelfHeatingUdVal_V_Set/1 -> Product/2

== system MDCC/DoCurCtr_sys/MDCC/SVM_Calc/DeadComp_Sys/DeadCur_Calc/N_Select_Calc/Subsystem1 ==
  Isd_A : Inport
  Isq_A : Inport  Port=2
  Add : Sum
  Constant : Constant  Value=2*pi  OutDataTypeStr=single
  Switch : Switch  Criteria=u2 > Threshold
  atan2 : mcbcontrolslib/atan2  outputUnit=Radians
      settings: SourceProductBaseCode=MT
  agIsE : Outport
  wires:
  Isd_A/1 -> atan2/2
  Isq_A/1 -> atan2/1
  atan2/1 -> Add/1, Switch/1, Switch/2
  Switch/1 -> agIsE/1
  Add/1 -> Switch/3
  Constant/1 -> Add/2

== system MDCC/DoCurCtr_sys/MDCC/SVM_Calc/DeadComp_Sys/DeadCur_Calc/N_Select_Calc/Subsystem2 ==
  eMtrSpd_rads : Inport
  eMtrPos_NULL : Inport  Port=2
  VfPwmFreq_Hz : Inport  Port=3
  Add : Sum  Inputs=+++
  Constant : Constant  Value=VuDeadCompen_agIPredAdpr_C
  Gain : Gain  Gain=2*pi/4095
  Gain1 : Gain  Gain=-1
  Gain2 : Gain  Gain=2*pi/4095
  Product : Product
  Subsystem : Subsystem
  Switch : Switch  Criteria=u2 > Threshold
  PreMtrPos : Outport
  wires:
  VfPwmFreq_Hz/1 -> Subsystem/1(VfPwmFreq_Hz)
  Subsystem/1(TimeComp) -> Product/2
  eMtrPos_NULL/1 -> Gain/1
  Product/1 -> Add/2
  Gain/1 -> Add/3
  Add/1 -> PreMtrPos/1
  eMtrSpd_rads/1 -> Product/1, Switch/2
  Constant/1 -> Gain2/1
  Gain1/1 -> Switch/3
  Gain2/1 -> Gain1/1, Switch/1
  Switch/1 -> Add/1

== system MDCC/DoCurCtr_sys/MDCC/SVM_Calc/DeadComp_Sys/DeadTime_Calc/Tavon_Calc/ia ==
  iPhase : Inport
  Phase_Dyc : Inport  Port=2
  uDcLink : Inport  Port=3
  Abs : Abs
  Add : Sum
  Compare To Constant : simulink/Logic and Bit Operations/Compare To Constant  relop=>  const=0  OutDataTypeStr=boolean
  If : If  IfExpression=u1 == 1
  If Action Subsystem : Subsystem  TreatAsAtomicUnit=on
  If Action Subsystem1 : Subsystem  TreatAsAtomicUnit=on
  Merge : Merge
  uDdeCalc : Subsystem
  uIgbtCalc : Subsystem
  "Duty_Avon " : Outport
  wires:
  iPhase/1 -> [C], Abs/1
  Abs/1 -> uIgbtCalc/1(iPhaseAbs), uDdeCalc/1(iPhaseAbs)
  uDdeCalc/1(uDde) -> [uDde]  "DeaduDde_U"
  uIgbtCalc/1(uIgbt) -> [uIgbt]  "DeaduIgbt_U"
  [C] -> Compare To Constant/1
  Compare To Constant/1 -> If/1
  If/1 -> If Action Subsystem/Action
  If/2 -> If Action Subsystem1/Action
  [uIgbt] -> If Action Subsystem1/2(uIgbt), If Action Subsystem/2(uIgbt)
  [uDde] -> If Action Subsystem1/3(uDde), If Action Subsystem/3(uDde)
  Phase_Dyc/1 -> Add/1, If Action Subsystem1/1(Phase_Dyc), If Action Subsystem/1(Phase_Dyc)
  uDcLink/1 -> If Action Subsystem/4(uDcLink), If Action Subsystem1/4(uDcLink)
  If Action Subsystem1/1("dycCorr ") -> Merge/2
  If Action Subsystem/1("dycCorr ") -> Merge/1
  Add/1 -> "Duty_Avon "/1
  Merge/1 -> Add/2

== system MDCC/DoCurCtr_sys/MDCC/SVM_Calc/DeadComp_Sys/DeadTime_Calc/Tavon_Calc/ib ==
  iPhase : Inport
  Phase_Dyc : Inport  Port=2
  uDcLink : Inport  Port=3
  Abs : Abs
  Add : Sum
  Compare To Constant : simulink/Logic and Bit Operations/Compare To Constant  relop=>  const=0  OutDataTypeStr=boolean
  If : If  IfExpression=u1 == 1
  If Action Subsystem : Subsystem  TreatAsAtomicUnit=on
  If Action Subsystem1 : Subsystem  TreatAsAtomicUnit=on
  Merge : Merge
  uDdeCalc : Subsystem
  uIgbtCalc : Subsystem
  "Duty_Avon " : Outport
  wires:
  iPhase/1 -> [C], Abs/1
  Abs/1 -> uIgbtCalc/1(iPhaseAbs), uDdeCalc/1(iPhaseAbs)
  uDdeCalc/1(uDde) -> [uDde]  "uDde_V"
  uIgbtCalc/1(uIgbt) -> [uIgbt]  "uIgbt_V"
  [C] -> Compare To Constant/1
  Compare To Constant/1 -> If/1
  If/1 -> If Action Subsystem/Action
  If/2 -> If Action Subsystem1/Action
  [uIgbt] -> If Action Subsystem1/2(uIgbt), If Action Subsystem/2(uIgbt)
  [uDde] -> If Action Subsystem1/3(uDde), If Action Subsystem/3(uDde)
  Phase_Dyc/1 -> Add/1, If Action Subsystem1/1(Phase_Dyc), If Action Subsystem/1(Phase_Dyc)
  uDcLink/1 -> If Action Subsystem/4(uDcLink), If Action Subsystem1/4(uDcLink)
  If Action Subsystem1/1("dycCorr ") -> Merge/2
  If Action Subsystem/1("dycCorr ") -> Merge/1
  Add/1 -> "Duty_Avon "/1
  Merge/1 -> Add/2

== system MDCC/DoCurCtr_sys/MDCC/SVM_Calc/DeadComp_Sys/DeadTime_Calc/Tavon_Calc/ic ==
  iPhase : Inport
  Phase_Dyc : Inport  Port=2
  uDcLink : Inport  Port=3
  Abs : Abs
  Add : Sum
  Compare To Constant : simulink/Logic and Bit Operations/Compare To Constant  relop=>  const=0  OutDataTypeStr=boolean
  If : If  IfExpression=u1 == 1
  If Action Subsystem : Subsystem  TreatAsAtomicUnit=on
  If Action Subsystem1 : Subsystem  TreatAsAtomicUnit=on
  Merge : Merge
  uDdeCalc : Subsystem
  uIgbtCalc : Subsystem
  "Duty_Avon " : Outport
  wires:
  iPhase/1 -> [C], Abs/1
  Abs/1 -> uIgbtCalc/1(iPhaseAbs), uDdeCalc/1(iPhaseAbs)
  uDdeCalc/1(uDde) -> [uDde]  "uDde_W"
  uIgbtCalc/1(uIgbt) -> [uIgbt]  "uIgbt_W"
  [C] -> Compare To Constant/1
  Compare To Constant/1 -> If/1
  If/1 -> If Action Subsystem/Action
  If/2 -> If Action Subsystem1/Action
  [uIgbt] -> If Action Subsystem1/2(uIgbt), If Action Subsystem/2(uIgbt)
  [uDde] -> If Action Subsystem1/3(uDde), If Action Subsystem/3(uDde)
  Phase_Dyc/1 -> Add/1, If Action Subsystem1/1(Phase_Dyc), If Action Subsystem/1(Phase_Dyc)
  uDcLink/1 -> If Action Subsystem/4(uDcLink), If Action Subsystem1/4(uDcLink)
  If Action Subsystem1/1("dycCorr ") -> Merge/2
  If Action Subsystem/1("dycCorr ") -> Merge/1
  Add/1 -> "Duty_Avon "/1
  Merge/1 -> Add/2

== system MDCC/DoCurCtr_sys/MDCC/SVM_Calc/MDSA/SVM_PU/N_Sector_calc/N_calc ==
  Uref1 : Inport
  Uref2 : Inport  Port=2
  Uref3 : Inport  Port=3
  Add : Sum  Inputs=+++
  ConstanT1 : Constant  Value=0  OutDataTypeStr=single
  Constant : Constant  OutDataTypeStr=single
  Gain : Gain
  Gain1 : Gain  Gain=2
  Gain2 : Gain  Gain=4
  Switch : Switch  Criteria=u2 > Threshold
  Switch1 : Switch  Criteria=u2 > Threshold
  Switch2 : Switch  Criteria=u2 > Threshold
  N_Sector : Outport
  wires:
  Uref1/1 -> Switch/2
  Uref2/1 -> Switch1/2
  Uref3/1 -> Switch2/2
  ConstanT1/1 -> Switch2/3, Switch/3, Switch1/3
  Constant/1 -> Switch2/1, Switch1/1, Switch/1
  Switch1/1 -> Gain1/1
  Switch/1 -> Gain/1
  Switch2/1 -> Gain2/1
  Add/1 -> N_Sector/1
  Gain/1 -> Add/1
  Gain1/1 -> Add/2
  Gain2/1 -> Add/3

== system MDCC/DoCurCtr_sys/MDCC/SVM_Calc/MDSA/SVM_PU/N_Sector_calc/Uref_Calc ==
  Ualpha : Inport
  Ubeta : Inport  Port=2
  Add : Sum  Inputs=+-
  Add1 : Sum  Inputs=--
  ConstanT1 : Constant  Value=sqrt(1)/2  OutDataTypeStr=single
  Constant : Constant  Value=sqrt(3)/2  OutDataTypeStr=single
  ProducT1 : Product
  Product : Product
  Signal Copy : SignalConversion  OverrideOpt=off
  Uref1 : Outport
  Uref2 : Outport  Port=2
  Uref3 : Outport  Port=3
  wires:
  Ubeta/1 -> ProducT1/1, Signal Copy/1
  Signal Copy/1 -> Uref1/1
  Ualpha/1 -> Product/1
  Constant/1 -> Product/2
  ConstanT1/1 -> ProducT1/2
  Product/1 -> Add1/1, Add/1
  ProducT1/1 -> Add1/2, Add/2
  Add/1 -> Uref2/1
  Add1/1 -> Uref3/1

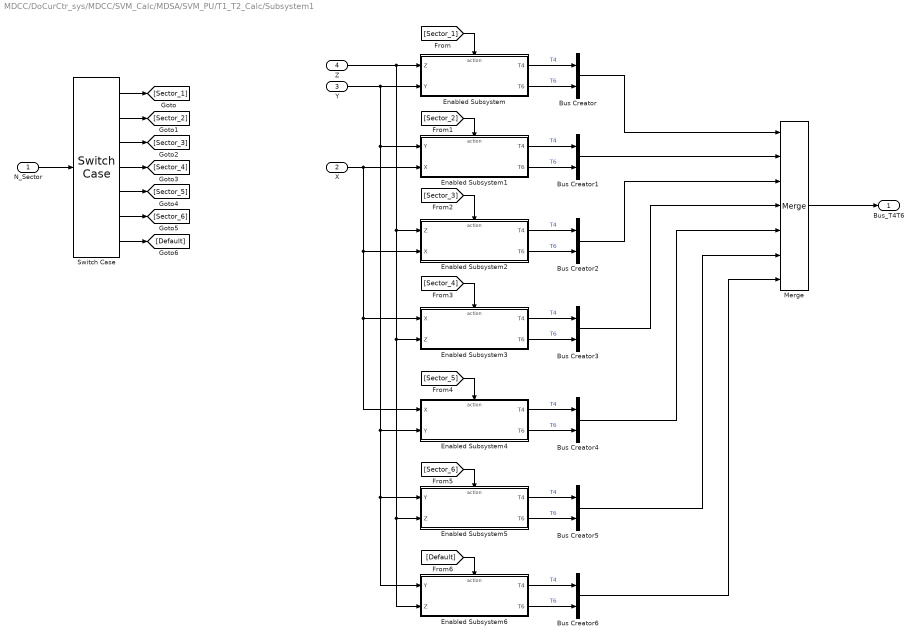
== system MDCC/DoCurCtr_sys/MDCC/SVM_Calc/MDSA/SVM_PU/T1_T2_Calc/Subsystem1 ==
  N_Sector : Inport
  X : Inport  Port=2
  Y : Inport  Port=3
  Z : Inport  Port=4
  Bus Creator{,1..6} (7 alike) : BusCreator  Inputs=2
  Enabled Subsystem : Subsystem  TreatAsAtomicUnit=on
  Enabled Subsystem1 : Subsystem  TreatAsAtomicUnit=on
  Enabled Subsystem2 : Subsystem  TreatAsAtomicUnit=on
  Enabled Subsystem3 : Subsystem  TreatAsAtomicUnit=on
  Enabled Subsystem4 : Subsystem  TreatAsAtomicUnit=on
  Enabled Subsystem5 : Subsystem  TreatAsAtomicUnit=on
  Enabled Subsystem6 : Subsystem  TreatAsAtomicUnit=on
  Merge : Merge  Inputs=7
  Switch Case : SwitchCase  CaseConditions={1,2,3,4,5,6}
  Bus_T4T6 : Outport
  wires:
  N_Sector/1 -> Switch Case/1
  Switch Case/1 -> [Sector_1]
  Switch Case/2 -> [Sector_2]
  Switch Case/3 -> [Sector_3]
  Switch Case/4 -> [Sector_4]
  Switch Case/5 -> [Sector_5]
  Switch Case/6 -> [Sector_6]
  Switch Case/7 -> [Default]
  [Sector_1] -> Enabled Subsystem/Action
  Y/1 -> Enabled Subsystem6/1(Y), Enabled Subsystem5/1(Y), Enabled Subsystem4/2(Y), Enabled Subsystem1/1(Y), Enabled Subsystem/2(Y)
  Z/1 -> Enabled Subsystem3/2(Z), Enabled Subsystem6/2(Z), Enabled Subsystem5/2(Z), Enabled Subsystem2/1(Z), Enabled Subsystem/1(Z)
  [Sector_2] -> Enabled Subsystem1/Action
  X/1 -> Enabled Subsystem4/1(X), Enabled Subsystem3/1(X), Enabled Subsystem2/2(X), Enabled Subsystem1/2(X)
  [Sector_3] -> Enabled Subsystem2/Action
  [Sector_4] -> Enabled Subsystem3/Action
  [Sector_5] -> Enabled Subsystem4/Action
  [Sector_6] -> Enabled Subsystem5/Action
  [Default] -> Enabled Subsystem6/Action
  Enabled Subsystem/1(T4) -> Bus Creator/1  "T4"
  Enabled Subsystem/2(T6) -> Bus Creator/2  "T6"
  Enabled Subsystem1/2(T6) -> Bus Creator1/2  "T6"
  Enabled Subsystem1/1(T4) -> Bus Creator1/1  "T4"
  Enabled Subsystem2/1(T4) -> Bus Creator2/1  "T4"
  Enabled Subsystem3/1(T4) -> Bus Creator3/1  "T4"
  Enabled Subsystem2/2(T6) -> Bus Creator2/2  "T6"
  Enabled Subsystem3/2(T6) -> Bus Creator3/2  "T6"
  Enabled Subsystem4/1(T4) -> Bus Creator4/1  "T4"
  Enabled Subsystem5/1(T4) -> Bus Creator5/1  "T4"
  Enabled Subsystem4/2(T6) -> Bus Creator4/2  "T6"
  Enabled Subsystem5/2(T6) -> Bus Creator5/2  "T6"
  Enabled Subsystem6/1(T4) -> Bus Creator6/1  "T4"
  Enabled Subsystem6/2(T6) -> Bus Creator6/2  "T6"
  Bus Creator/1 -> Merge/1
  Bus Creator1/1 -> Merge/2
  Bus Creator2/1 -> Merge/3
  Bus Creator3/1 -> Merge/4
  Bus Creator4/1 -> Merge/5
  Bus Creator5/1 -> Merge/6
  Bus Creator6/1 -> Merge/7
  Merge/1 -> Bus_T4T6/1

== system MDCC/DoCurCtr_sys/MDCC/SVM_Calc/MDSA/SVM_PU/T1_T2_Calc/Subsystem2 ==
  Bus_T4T6 : Inport
  Add : Sum
  Bus Selector : BusSelector  OutputSignals=T4,T6
  Bus_T4T1 : InportShadow
  Bus_T4T2 : InportShadow
  Bus_T4T3 : InportShadow
  If : If  IfExpression=u1 > 1.154  ElseIfExpressions=u1 > 1
  If Action Subsystem : Subsystem  TreatAsAtomicUnit=on
  If Action Subsystem1 : Subsystem  TreatAsAtomicUnit=on
  If Action Subsystem2 : Subsystem  TreatAsAtomicUnit=on
  Merge : Merge  Inputs=3
  Merge1 : Merge  Inputs=3
  T1 : Outport
  T2 : Outport  Port=2
  wires:
  Bus_T4T6/1 -> Bus Selector/1
  Bus Selector/1 -> Add/1  "<T4>"
  Bus Selector/2 -> Add/2  "<T6>"
  Add/1 -> If/1
  If/3 -> If Action Subsystem/Action
  If/2 -> If Action Subsystem1/Action
  If/1 -> If Action Subsystem2/Action
  Bus_T4T1/1 -> If Action Subsystem/1(Bus_T4T6)
  Bus_T4T2/1 -> If Action Subsystem1/1(Bus_T4T6)
  Bus_T4T3/1 -> If Action Subsystem2/1(Bus_T4T6)
  Merge/1 -> T1/1
  If Action Subsystem2/1(T1) -> Merge/1
  If Action Subsystem1/1(T1) -> Merge/2
  If Action Subsystem/1(T1) -> Merge/3
  If Action Subsystem2/2(T2) -> Merge1/1
  If Action Subsystem1/2(T2) -> Merge1/2
  If Action Subsystem/2(T2) -> Merge1/3
  Merge1/1 -> T2/1

== system MDCC/DoCurCtr_sys/MDCC/SVM_Calc/MDSA/SVM_PU/T1_T2_Calc/T4_T6 ==
  T4 : Inport
  T6 : Inport  Port=2
  Add : Sum
  Divide : Product  Inputs=*/
  Divide1 : Product  Inputs=*/
  Mux : Mux  Inputs=2
  Mux1 : Mux  Inputs=2
  Switch : Switch  Criteria=u2 > Threshold  Threshold=1
  T4_T6 : Outport
  wires:
  T4/1 -> Add/1, Mux1/1, Divide/1
  T6/1 -> Mux1/2, Add/2, Divide1/1
  Add/1 -> Divide1/2, Divide/2, Switch/2
  Divide/1 -> Mux/1  "T4"
  Divide1/1 -> Mux/2  "T6"
  Mux/1 -> Switch/1
  Mux1/1 -> Switch/3
  Switch/1 -> T4_T6/1

== system MDCC/DoCurCtr_sys/MDCC/SVM_Calc/MDSA/SVM_PU/Tcm_Calc/If Action Subsystem ==
  Ta : Inport
  Tb : Inport  Port=2
  Tc : Inport  Port=3
  Action Port : ActionPort  ActionPortLabel=case [ 1 ]:
  Tcm1 : Outport
  Tcm2 : Outport  Port=2
  Tcm3 : Outport  Port=3
  wires:
  Tb/1 -> Tcm1/1
  Ta/1 -> Tcm2/1
  Tc/1 -> Tcm3/1

== system MDCC/DoCurCtr_sys/MDCC/SVM_Calc/MDSA/SVM_PU/Tcm_Calc/If Action Subsystem1 ==
  Ta : Inport
  Tb : Inport  Port=2
  Tc : Inport  Port=3
  Action Port : ActionPort  ActionPortLabel=case [ 3 ]:
  Tcm1 : Outport
  Tcm2 : Outport  Port=2
  Tcm3 : Outport  Port=3
  wires:
  Ta/1 -> Tcm1/1
  Tb/1 -> Tcm2/1
  Tc/1 -> Tcm3/1

== system MDCC/DoCurCtr_sys/MDCC/SVM_Calc/MDSA/SVM_PU/Tcm_Calc/If Action Subsystem2 ==
  Ta : Inport
  Tb : Inport  Port=2
  Tc : Inport  Port=3
  Action Port : ActionPort  ActionPortLabel=case [ 4 ]:
  Tcm1 : Outport
  Tcm2 : Outport  Port=2
  Tcm3 : Outport  Port=3
  wires:
  Tc/1 -> Tcm1/1
  Tb/1 -> Tcm2/1
  Ta/1 -> Tcm3/1

== system MDCC/DoCurCtr_sys/MDCC/SVM_Calc/MDSA/SVM_PU/Tcm_Calc/If Action Subsystem3 ==
  Ta : Inport
  Tb : Inport  Port=2
  Tc : Inport  Port=3
  Action Port : ActionPort  ActionPortLabel=case [ 5 ]:
  Tcm1 : Outport
  Tcm2 : Outport  Port=2
  Tcm3 : Outport  Port=3
  wires:
  Tc/1 -> Tcm1/1
  Tb/1 -> Tcm3/1
  Ta/1 -> Tcm2/1

== system MDCC/DoCurCtr_sys/MDCC/SVM_Calc/MDSA/SVM_PU/Tcm_Calc/If Action Subsystem4 ==
  Ta : Inport
  Tb : Inport  Port=2
  Tc : Inport  Port=3
  Action Port : ActionPort  ActionPortLabel=case [ 6 ]:
  Tcm1 : Outport
  Tcm2 : Outport  Port=2
  Tcm3 : Outport  Port=3
  wires:
  Tc/1 -> Tcm2/1
  Tb/1 -> Tcm1/1
  Ta/1 -> Tcm3/1

== system MDCC/DoCurCtr_sys/MDCC/SVM_Calc/MDSA/SVM_PU/Tcm_Calc/If Action Subsystem5 ==
  Ta : Inport
  Tb : Inport  Port=2
  Tc : Inport  Port=3
  Action Port : ActionPort  ActionPortLabel=default:
  Tcm1 : Outport
  Tcm2 : Outport  Port=2
  Tcm3 : Outport  Port=3
  wires:
  Tc/1 -> Tcm2/1
  Tb/1 -> Tcm1/1
  Ta/1 -> Tcm3/1

== system MDCC/DoCurCtr_sys/MDCC/SVM_Calc/MDSA/SVM_PU/Tcm_Calc/If Action Subsystem7 ==
  Ta : Inport
  Tb : Inport  Port=2
  Tc : Inport  Port=3
  Action Port : ActionPort  ActionPortLabel=case [ 2 ]:
  Tcm1 : Outport
  Tcm2 : Outport  Port=2
  Tcm3 : Outport  Port=3
  wires:
  Ta/1 -> Tcm1/1
  Tc/1 -> Tcm2/1
  Tb/1 -> Tcm3/1

== system MDCC/DoCurCtr_sys/MDCC/SVM_Calc/MDSA/SVPWM/vIntp_PWMFOC_CalSec/CalABC ==
  Bus_Vabc_IN : Inport
  Bus Creator : BusCreator  Inputs=3
  Bus Selector : BusSelector  OutputSignals=Va,Vb,Vc
  CalA : Subsystem
  CalB : Subsystem
  CalC : Subsystem
  Bus_ABC : Outport
  wires:
  Bus Creator/1 -> Bus_ABC/1
  CalA/1(A) -> Bus Creator/1  "A"
  CalC/1(C) -> Bus Creator/3  "C"
  CalB/1(B) -> Bus Creator/2  "B"
  Bus Selector/3 -> CalC/1(In1)  "<Vc>"
  Bus Selector/2 -> CalB/1(In1)  "<Vb>"
  Bus Selector/1 -> CalA/1(In1)  "<Va>"
  Bus_Vabc_IN/1 -> Bus Selector/1

== system MDCC/DoCurCtr_sys/MDCC/SVM_Calc/MDSA/SVPWM/vIntp_PWMFOC_CalSec/CalSecValue ==
  Bus_ABC_IN : Inport
  Add : Sum  Inputs=+++
  Bus Selector : BusSelector  OutputSignals=A,B,C
  Constant : Constant  Value=2
  Constant1 : Constant  Value=4
  Data Type Conversion : DataTypeConversion
  Data Type Conversion1 : DataTypeConversion
  Data Type Conversion2 : DataTypeConversion  OutDataTypeStr=uint8
  Data Type Conversion3 : DataTypeConversion  OutDataTypeStr=uint8
  Data Type Conversion4 : DataTypeConversion  OutDataTypeStr=uint8
  Lookup_Table : LookupNDDirect  NumberOfTableDimensions=1  Table=[2,2,6,1,4,3,5]  TableDataTypeStr=uint8
      settings: AttributesFormatString=-------------------------------\nTable: %<Table>
  Product : Product
  Product1 : Product
  SecValue : Outport
  N_VALUE : Outport  Port=2
  wires:
  Data Type Conversion4/1 -> Add/3
  Data Type Conversion3/1 -> Add/2
  Lookup_Table/1 -> SecValue/1
  Data Type Conversion2/1 -> Lookup_Table/1, N_VALUE/1
  Add/1 -> Data Type Conversion2/1
  Product1/1 -> Data Type Conversion4/1
  Product/1 -> Data Type Conversion3/1
  Bus Selector/1 -> Add/1  "<A>"
  Bus Selector/3 -> Product1/1  "<C>"
  Bus Selector/2 -> Product/1  "<B>"
  Data Type Conversion1/1 -> Product1/2
  Data Type Conversion/1 -> Product/2
  Constant1/1 -> Data Type Conversion1/1
  Constant/1 -> Data Type Conversion/1
  Bus_ABC_IN/1 -> Bus Selector/1

== system MDCC/DoCurCtr_sys/MDCC/SVM_Calc/MDSA/SVPWM/vIntp_PWMFOC_CalSec/CalVaVbVc ==
  Bus_UalphaUbeta : Inport
  Bus Creator : BusCreator  Inputs=3
  CalVa : Subsystem
  CalVb : Subsystem
  CalVc : Subsystem
  Bus_Vabc : Outport
  wires:
  Bus Creator/1 -> Bus_Vabc/1
  CalVa/1(Va) -> Bus Creator/1  "Va"
  CalVc/1(Vc) -> Bus Creator/3  "Vc"
  CalVb/1(Vb) -> Bus Creator/2  "Vb"
  Bus_UalphaUbeta/1 -> CalVa/1(In1), CalVb/1(In1), CalVc/1(In1)

== system MDCC/DoCurCtr_sys/MDCC/SVM_Calc/MDSA/SVPWM/vIntp_PWMFOC_CalTriCompValue/CalCMPValue ==
  Bus_Tabc_IN : Inport
  N_VALUE_IN : Inport  Port=2
  Merge : Merge  Inputs=6
  Sec1 : Subsystem
  Sec2 : Subsystem
  Sec3 : Subsystem
  Sec4 : Subsystem
  Sec5 : Subsystem
  Sec6 : Subsystem
  Switch Case : SwitchCase  CaseConditions={1,2,3,4,5,6}  ShowDefaultCase=off
  Bus_CMP : Outport
  wires:
  Sec1/1(Bus_CMP) -> Merge/1
  Sec6/1(Bus_CMP) -> Merge/6
  Sec2/1(Bus_CMP) -> Merge/2
  Sec5/1(Bus_CMP) -> Merge/5
  Sec3/1(Bus_CMP) -> Merge/3
  Sec4/1(Bus_CMP) -> Merge/4
  [sec6] -> Sec6/Action
  [sec5] -> Sec5/Action
  [sec4] -> Sec4/Action
  [sec3] -> Sec3/Action
  [sec2] -> Sec2/Action
  [sec1] -> Sec1/Action
  Switch Case/6 -> [sec6]
  Switch Case/5 -> [sec5]
  Switch Case/4 -> [sec4]
  Switch Case/3 -> [sec3]
  Switch Case/2 -> [sec2]
  Switch Case/1 -> [sec1]
  Merge/1 -> Bus_CMP/1
  Bus_Tabc_IN/1 -> Sec1/1(Bus_Tabc_IN), Sec3/1(Bus_Tabc_IN), Sec5/1(Bus_Tabc_IN), Sec6/1(Bus_Tabc_IN), Sec4/1(Bus_Tabc_IN), Sec2/1(Bus_Tabc_IN)
  N_VALUE_IN/1 -> Switch Case/1

== system MDCC/DoCurCtr_sys/MDCC/SVM_Calc/MDSA/SVPWM/vIntp_PWMFOC_CalTriCompValue/CalTabc ==
  Bus_XYZ_IN : Inport
  Bus_Ts_Vdc : Inport  Port=2
  N_VALUE_IN : Inport  Port=3
  Cal_T1T2 : Subsystem
  Cal_TabcValue : Subsystem
  Bus_Tabc : Outport
  wires:
  Cal_TabcValue/1(Bus_Tabc) -> Bus_Tabc/1
  Cal_T1T2/1(Bus_T1T2_OUT) -> Cal_TabcValue/1(Bus_T1T2_IN)
  N_VALUE_IN/1 -> Cal_T1T2/2(N_VALUE_IN)
  Bus_XYZ_IN/1 -> Cal_T1T2/1(Bus_XYZ_IN)
  Bus_Ts_Vdc/1 -> Cal_TabcValue/2(Bus_Ts_Vdc)

== system MDCC/DoCurCtr_sys/MDCC/SVM_Calc/MDSA/SVPWM/vIntp_PWMFOC_CalTriCompValue/CalXYZ ==
  Bus_UalphaUbeta : Inport
  Bus_Ts_Vdc : Inport  Port=2
  Bus Creator : BusCreator  Inputs=3
  Cal_X : Subsystem
  Cal_Y : Subsystem
  Cal_Z : Subsystem
  BUS_XYZ : Outport
  wires:
  Bus_Ts_Vdc/1 -> Cal_Y/2(Bus_Ts_Vdc), Cal_X/2(Bus_Ts_Vdc), Cal_Z/2(Bus_Ts_Vdc)
  Bus Creator/1 -> BUS_XYZ/1
  Cal_Z/1(Z_Value) -> Bus Creator/3  "Z"
  Cal_X/1(X_Value) -> Bus Creator/1  "X"
  Cal_Y/1(Y_Value) -> Bus Creator/2  "Y"
  Bus_UalphaUbeta/1 -> Cal_X/1(Bus_UalphaUbeta), Cal_Y/1(Bus_UalphaUbeta), Cal_Z/1(Bus_UalphaUbeta)

== system MDCC/DoCurCtr_sys/MDCC/UdUqCalc_Sys/MDCC_MCF_Sys/Enabled Subsystem/Harmonic_Injection_11/Set_11_steps_current_isdqdes ==
  TDC_TrqDesFlt : Inport
  1-D Lookup Table : Lookup_n-D  NumberOfTableDimensions=1  BreakpointsForDimension1=KfMDCC_MCF_HarmIn1113ZRY_Trq_Nm  Table=KfMDCC_MCF_HarmIn11ZRY_Isd_A  InternalRulePriority=Speed  RndMeth=Simplest  InputSameDT=on
  1-D Lookup Table1 : Lookup_n-D  NumberOfTableDimensions=1  BreakpointsForDimension1=KfMDCC_MCF_HarmIn1113ZRY_Trq_Nm  Table=KfMDCC_MCF_HarmIn11ZRY_Isq_A  InternalRulePriority=Speed  RndMeth=Simplest  InputSameDT=on
  Bus Creator1 : BusCreator  Inputs=2
  Bus Creator2 : BusCreator  Inputs=2
  Bus Selector1 : BusSelector  OutputSignals=MCF_IsdDes11Harm_A,MCF_IsqDes11Harm_A
  CAL_MCF_IsDes11Harm_f32 : Constant  Value=KfMDCC_MCF_IsDes11Harm_A
  CAL_MCF_IsThetaDes11Harm_f32 : Constant  Value=KfMDCC_MCF_IsThetaDes11Harm_NULL
  CAL_MCF_flgHarmInIsdqTab11ZR_b : Constant  Value=KbMDCC_MCF_flgHarmInIsdqTab11ZR_flg
  LookUpEAngleCosSin1 : Subsystem  TreatAsAtomicUnit=on  RTWFcnName=MCF_MDCC_LookUpEAngleCosSin  RTWFileName=MDCC
      settings: RTWFcnNameOpts=User specified
  Product11 : Product  OutDataTypeStr=uint16
  Product2 : Product
  Product5 : Product
  Signal Copy : SignalConversion  OverrideOpt=off
  Signal Copy1 : SignalConversion  OverrideOpt=off
  Sine_and_cosine_table1 : Constant  Value=11.31111  OutDataTypeStr=single
  Switch1 : Switch  Criteria=u2 ~= 0
  VfMDCC_MCF_IsdDes11Harm_A : Outport  VectorParamsAs1DForOutWhenUnconnected=off
  VfMDCC_MCF_IsqDes11Harm_A : Outport  Port=2  VectorParamsAs1DForOutWhenUnconnected=off
  wires:
  Signal Copy1/1 -> VfMDCC_MCF_IsqDes11Harm_A/1  "VfMDCC_MCF_IsqDes11Harm_A"
  Signal Copy/1 -> VfMDCC_MCF_IsdDes11Harm_A/1  "VfMDCC_MCF_IsdDes11Harm_A"
  Bus Selector1/2 -> Signal Copy1/1  "<MCF_IsqDes11Harm_A>"
  Bus Selector1/1 -> Signal Copy/1  "<MCF_IsdDes11Harm_A>"
  Switch1/1 -> Bus Selector1/1
  CAL_MCF_flgHarmInIsdqTab11ZR_b/1 -> Switch1/2
  1-D Lookup Table1/1 -> Bus Creator2/2  "MCF_IsqDes11Harm_A"
  Bus Creator2/1 -> Switch1/1
  1-D Lookup Table/1 -> Bus Creator2/1  "MCF_IsdDes11Harm_A"
  TDC_TrqDesFlt/1 -> 1-D Lookup Table/1, 1-D Lookup Table1/1
  CAL_MCF_IsDes11Harm_f32/1 -> Product5/1, Product2/1
  Sine_and_cosine_table1/1 -> Product11/2
  LookUpEAngleCosSin1/2(VfMDCC_EAngleSin_NULL) -> Product5/2
  Product2/1 -> Bus Creator1/1  "MCF_IsdDes11Harm_A"
  Bus Creator1/1 -> Switch1/3
  Product11/1 -> LookUpEAngleCosSin1/1(VuMDCC_MotorPositionCnt_NULL)
  CAL_MCF_IsThetaDes11Harm_f32/1 -> Product11/1
  Product5/1 -> Bus Creator1/2  "MCF_IsqDes11Harm_A"
  LookUpEAngleCosSin1/1(VfMDCC_EAngleCos_NULL) -> Product2/2
